simulink model "Single_Phase_Half_Wave_Rectifier_RL_FWD_Load"  (R2022b)
settings: Solver=ode23t  StartTime=0.0  StopTime=.1  MaxStep=1e-5  RelTol=1e-3
libraries: spsCurrentMeasurementLib x3, spsDiodeLib x2, spsVoltageMeasurementLib x2, spsACVoltageSourceLib x1, spsSeriesRLCBranchLib x1, spspowerguiLib x1
settings Model: Creator=Ahmed Aboeita  LastModifiedBy=Ahmed Aboeita

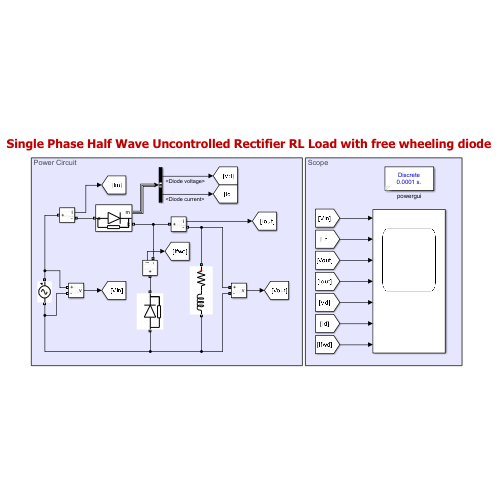
[thumbnail: Simulink's stored preview of the top-level diagram]
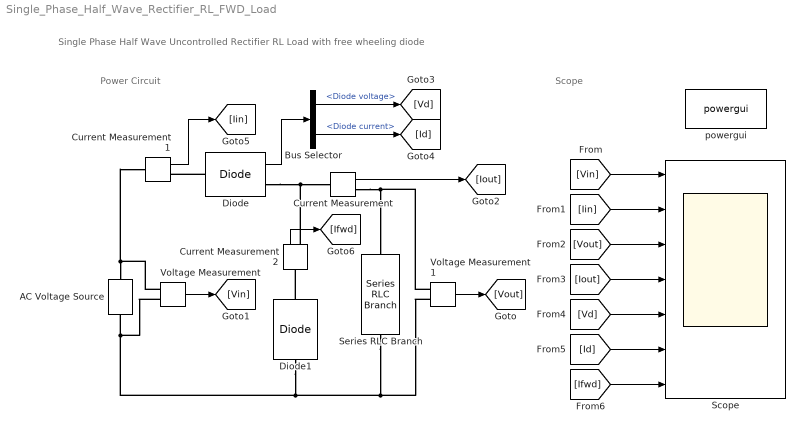
== system Single_Phase_Half_Wave_Rectifier_RL_FWD_Load ==
  note: Single Phase Half Wave Uncontrolled Rectifier RL Load with free wheeling diode
  note: Power Circuit
  note: Scope
  AC Voltage Source : spsACVoltageSourceLib/AC Voltage Source  Amplitude=100  Phase=0  Frequency=50  SampleTime=0  Measurements=None  BusType=swing  Pref=10e3  Qref=0  Qmin=-inf  Qmax=+inf
  Bus Selector : BusSelector  OutputSignals=Diode voltage,Diode current
  Current Measurement : spsCurrentMeasurementLib/Current Measurement  PhasorSimulation=off  OutputType=Complex  PSBequivalent=0
  Current Measurement1 : spsCurrentMeasurementLib/Current Measurement  PhasorSimulation=off  OutputType=Complex  PSBequivalent=0
  Current Measurement2 : spsCurrentMeasurementLib/Current Measurement  PhasorSimulation=off  OutputType=Complex  PSBequivalent=0
  Diode : spsDiodeLib/Diode  Ron=0.001  Lon=0  Vf=0.8  IC=0  UseSnubber=0  Rs=500  Cs=250e-9  Measurements=on
  Diode1 : spsDiodeLib/Diode  Ron=0.001  Lon=0  Vf=0.8  IC=0  UseSnubber=0  Rs=500  Cs=250e-9  Measurements=off
  Scope : Scope  NumInputPorts=7
  Series RLC Branch : spsSeriesRLCBranchLib/Series RLC Branch  LConnTagsString=__new0  RConnTagsString=__new0  BranchType=RL  Resistance=50  Inductance=200e-3  SetiL0=off  InitialCurrent=0  Capacitance=1e-6  Setx0=off  InitialVoltage=0  Measurements=None
  Voltage Measurement : spsVoltageMeasurementLib/Voltage Measurement  PhasorSimulation=off  OutputType=Complex  PSBequivalent=0
  Voltage Measurement1 : spsVoltageMeasurementLib/Voltage Measurement  PhasorSimulation=off  OutputType=Complex  PSBequivalent=0
  powergui : spspowerguiLib/powergui  Priority=1  SimulationMode=Discrete  SampleTime=1e-4  frequency=60  Iterations=50  frequencyindice=50  Pbase=100e6  ErrMax=1e-4  UnitsV=kV  UnitsW=MW  buscounter=0  FunctionMessages=off  echomessages=off  EnableUseOfTLC=off  CurrentSourceSwitches=off  DisableSnubberDevices=off  DisableRonSwitches=off  DisableVfSwitches=off  DisplayEquations=off  AutomaticDiscreteSolvers=off  SolverType=Tustin/Backward Euler (TBE)  Interpol=off  ExternalGateDelay=off  methode=off  Ts=100  x0status=blocks  SPID=on  SwTol=0  HookPort=off  NonlinearTolerance=1e-4  nMaxIteration=100  ContinueOnMaxIteration=off  RestoreLinks=warning  ResistiveCurrentMeasurement=off  Frange=[0:2:500]  Ylog=off  Xlog=on  ShowGrid=off  save=off  variable=ZData  structure=0  ZoomFFT=off  StartTime=0.0  cycles=1  DisplayStyle=1  fundamental=60  FreqAxis=off  MaxFrequency=1000  frequencyindicesteady=1  RmsSteady=1  display=off
  wires:
  Voltage Measurement1/1 -> [Vout]
  Voltage Measurement/1 -> [Vin]
  Current Measurement/1 -> [Iout]
  Diode/1 -> Bus Selector/1
  Bus Selector/1 -> [Vd]  "<Diode voltage>"
  Bus Selector/2 -> [Id]  "<Diode current>"
  [Vin] -> Scope/1
  Current Measurement1/1 -> [Iin]
  [Iin] -> Scope/2
  [Id] -> Scope/6
  [Vout] -> Scope/3
  [Iout] -> Scope/4
  [Vd] -> Scope/5
  Current Measurement2/1 -> [Ifwd]
  [Ifwd] -> Scope/7
  connections:
  Voltage Measurement/LConn1 -- Current Measurement1/LConn1 -- AC Voltage Source/RConn1
  Voltage Measurement1/LConn1 -- Series RLC Branch/LConn1 -- Current Measurement/RConn1
  Series RLC Branch/RConn1 -- Voltage Measurement1/LConn2 -- Diode1/LConn1 -- Voltage Measurement/LConn2 -- AC Voltage Source/LConn1
  Diode/RConn1 -- Current Measurement2/RConn1 -- Current Measurement/LConn1
  Diode/LConn1 -- Current Measurement1/RConn1
  Diode1/RConn1 -- Current Measurement2/LConn1
